simulink model "Torque_Rod_Sim"  (R2024a)
settings: Solver=VariableStepAuto  StartTime=0.0  StopTime=10.0  RelTol=1e-3
libraries: simulink x1
settings Model: Creator=RAJDEEP PAUL  LastModifiedBy=RAJDEEP PAUL

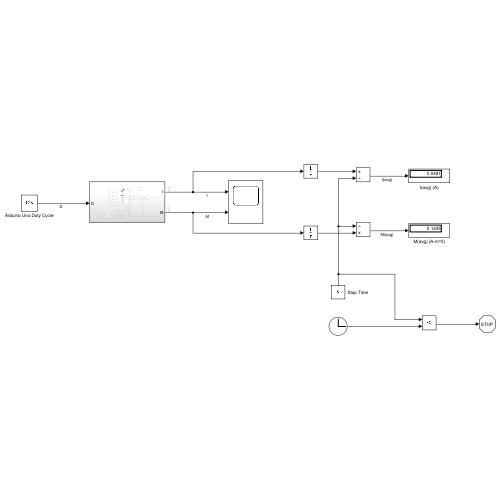
[thumbnail: Simulink's stored preview of the top-level diagram]
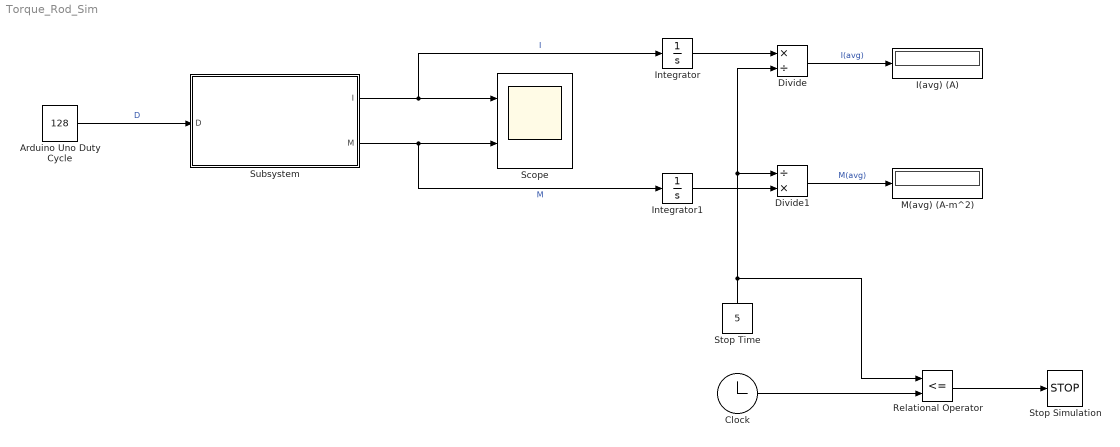
== system Torque_Rod_Sim ==
  Arduino Uno Duty Cycle : Constant  Value=128
  Clock : Clock
  Divide : Product  Inputs=*/
  Divide1 : Product  Inputs=/*
  I(avg) (A) : Display
  Integrator : Integrator
  Integrator1 : Integrator
  M(avg) (A-m^2) : Display
  Relational Operator : RelationalOperator  Operator=<=  OutDataTypeStr=boolean  RndMeth=Simplest  InputSameDT=off
  Scope : Scope  NumInputPorts=2
  Stop Simulation : Stop
  Stop Time : Constant  Value=5
  Subsystem : Subsystem
  wires:
  Arduino Uno Duty Cycle/1 -> Subsystem/1(D)  "D"
  Subsystem/1(I) -> Integrator/1, Scope/1  "I"
  Subsystem/2(M) -> Integrator1/1, Scope/2  "M"
  Integrator/1 -> Divide/1
  Integrator1/1 -> Divide1/2
  Stop Time/1 -> Relational Operator/1, Divide/2, Divide1/1
  Divide/1 -> I(avg) (A)/1  "I(avg)"
  Divide1/1 -> M(avg) (A-m^2)/1  "M(avg)"
  Clock/1 -> Relational Operator/2
  Relational Operator/1 -> Stop Simulation/1

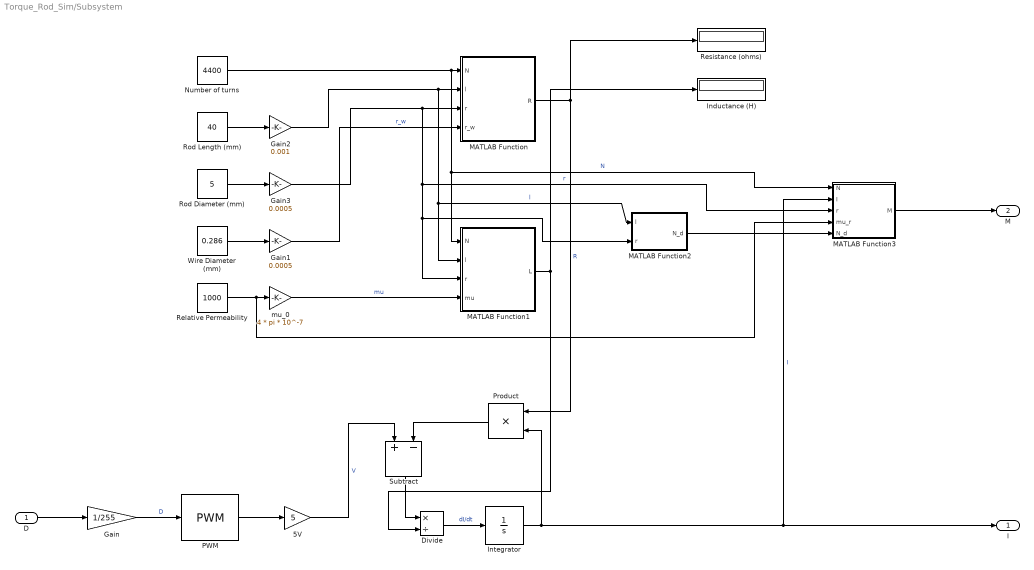
== system Torque_Rod_Sim/Subsystem ==
  D : Inport
  5V : Gain  Gain=5
  Divide : Product  Inputs=*/
  Gain : Gain  Gain=1/255
  Gain1 : Gain  Gain=0.0005
  Gain2 : Gain  Gain=0.001
  Gain3 : Gain  Gain=0.0005
  Inductance (H) : Display
  Integrator : Integrator
  MATLAB Function : MATLAB Function  TreatAsAtomicUnit=on
  MATLAB Function1 : MATLAB Function  TreatAsAtomicUnit=on
  MATLAB Function2 : MATLAB Function  TreatAsAtomicUnit=on
  MATLAB Function3 : MATLAB Function  TreatAsAtomicUnit=on
  Number of turns : Constant  Value=4400
  PWM : simulink/Discontinuities/PWM  DisableCoverage=on  Period=1/490  InitialDelay=0  DisallowZeroDutyCycle=off  RunAtFixedTimeIntervals=off  SampleTime=0.1
  Product : Product
  Relative Permeability : Constant  Value=1000
  Resistance (ohms) : Display
  Rod Diameter (mm) : Constant  Value=5
  Rod Length (mm) : Constant  Value=40
  Subtract : Sum  Inputs=+-
  Wire Diameter (mm) : Constant  Value=0.286
  mu_0 : Gain  Gain=4 * pi * 10^-7
  I : Outport
  M : Outport  Port=2
  wires:
  D/1 -> Gain/1
  Gain/1 -> PWM/1  "D"
  PWM/1 -> 5V/1
  Wire Diameter (mm)/1 -> Gain1/1
  Rod Length (mm)/1 -> Gain2/1
  Rod Diameter (mm)/1 -> Gain3/1
  Number of turns/1 -> MATLAB Function1/1(N), MATLAB Function3/1(N), MATLAB Function/1(N)  "N"
  Gain1/1 -> MATLAB Function/4(r_w)  "r_w"
  Gain2/1 -> MATLAB Function1/2(l), MATLAB Function2/1(l), MATLAB Function/2(l)  "l"
  Gain3/1 -> MATLAB Function1/3(r), MATLAB Function2/2(r), MATLAB Function3/3(r), MATLAB Function/3(r)  "r"
  Relative Permeability/1 -> MATLAB Function3/4(mu_r), mu_0/1
  mu_0/1 -> MATLAB Function1/4(mu)  "mu"
  Integrator/1 -> MATLAB Function3/2(I), I/1, Product/2  "I"
  MATLAB Function/1(R) -> Resistance (ohms)/1, Product/1  "R"
  Product/1 -> Subtract/2
  5V/1 -> Subtract/1  "V"
  Subtract/1 -> Divide/1
  MATLAB Function1/1(L) -> Divide/2, Inductance (H)/1
  Divide/1 -> Integrator/1  "dI/dt"
  MATLAB Function2/1(N_d) -> MATLAB Function3/5(N_d)
  MATLAB Function3/1(M) -> M/1

== matlab function Torque_Rod_Sim/Subsystem/MATLAB Function1 ==
  data: N input; l input; r input; L output; mu input
function L = fcn(N, l, r, mu)

L = (mu * N^2 * pi * r^2) / l;

== matlab function Torque_Rod_Sim/Subsystem/MATLAB Function ==
  data: N input; l input; r input; R output; r_w input
function R = fcn(N, l, r, r_w)

l_w = 0;
N_layer = fix(l / (2 * r_w));
layers = fix(N / N_layer);

for i = 0 : layers - 1

    l_w = l_w + (N_layer * 2 * pi * (r + (2 * i + 1) * r_w));

end

e = 1.7 * 10^-8;

R = (e * l_w) / (pi * r_w^2);

== matlab function Torque_Rod_Sim/Subsystem/MATLAB Function2 ==
  data: l input; N_d output; r input
function N_d = fcn(l, r)

x = l / r;

N_d = (4 * (log(x) - 1)) / (x^2 - 4 * log(x));

== matlab function Torque_Rod_Sim/Subsystem/MATLAB Function3 ==
  data: N input; M output; I input; r input; mu_r input; N_d input
function M = fcn(N, I, r, mu_r, N_d)

K = 1 + (mu_r - 1) / (1 + N_d * (mu_r - 1));

M = N * I * pi * r^2 * K;
